simulink model "B_dot_filter"  (R2023a)
settings: Solver=ode45  StartTime=0.0  StopTime=48000.0  RelTol=1e-3  EnableMultiTasking=on
libraries: aausat3_lib x5
settings Model: NumberOfSteps=1000  Creator=KFJensen  LastModifiedBy=jacobel-omar
settings SolverCC: AlgebraicLoopSolver=TrustRegion
settings DataIOCC: SaveFormat=Array  SignalLoggingSaveFormat=ModelDataLogs  ReturnWorkspaceOutputs=off
settings OptimizationCC: DefaultParameterBehavior=Inlined  ExpressionDepthLimit=2147483647  LifeSpan=inf  SimCompilerOptimization=on
settings DebuggingCC: SignalInfNanChecking=error  UnderspecifiedInitializationDetection=Classic  MergeDetectMultiDrivingBlocksExec=none  SolverPrmCheckMsg=warning  IntegerOverflowMsg=error  ParameterUnderflowMsg=error  FcnCallInpInsideContextMsg=warning  UnconnectedInputMsg=warning  UnconnectedOutputMsg=warning  UnconnectedLineMsg=warning  AssertControl=DisableAll  StateNameClashWarn=warning  SFUnexpectedBacktrackingDiag=warning  SFNoUnconditionalDefaultTransitionDiag=warning  SFExecutionAtInitializationDiag=none  IntegerSaturationMsg=error  ArithmeticOperatorsInVariantConditions=warning
settings HardwareCC: ProdBitPerPointer=32  ProdBitPerSizeT=32  ProdBitPerPtrDiffT=32  ProdLargestAtomicFloat=None  ProdIntDivRoundTo=Undefined  ProdEndianess=Unspecified  ProdWordSize=32  ProdHWDeviceType=Generic->Unspecified (assume 32-bit Generic)
settings ModelReferenceCC: PropagateSignalLabelsOutOfModel=off
settings SFSimCC: SimUseLocalCustomCode=off  SimParseCustomCode=off  CustomCodeUndefinedFunction=UseInterfaceOnly
settings RTWCC: RTWUseLocalCustomCode=off
settings CodeAppCC: StateflowObjectComments=on
settings GRTTargetCC: TargetLangStandard=C89/C90 (ANSI)  CombineOutputUpdateFcns=off  GRTInterface=on
settings ConfigComp: CovMetricSettings=dw  CovSaveCumulativeToWorkspaceVar=on  CovSaveSingleToWorkspaceVar=on  CovExternalEMLEnable=off

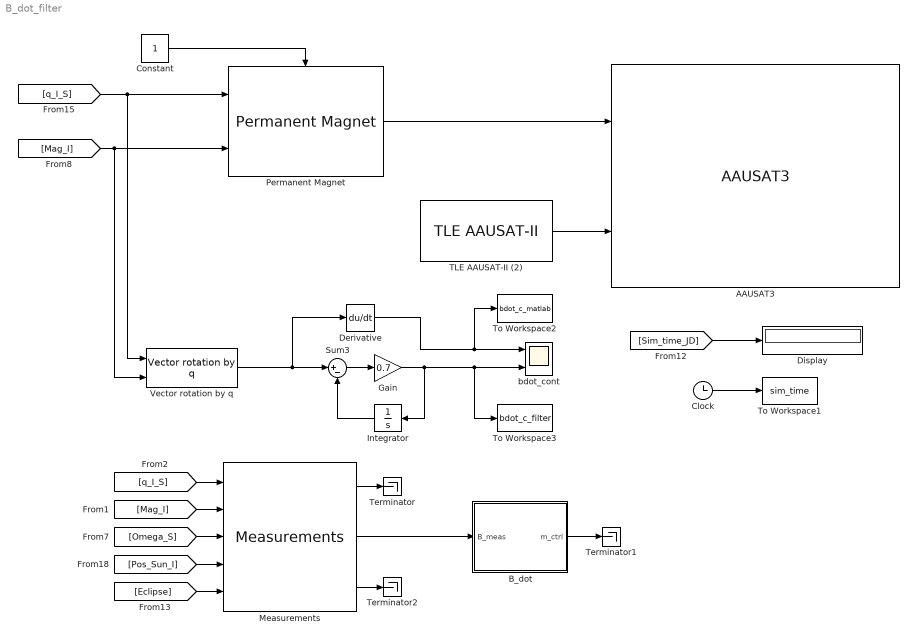
== system B_dot_filter ==
  AAUSAT3 : aausat3_lib/AAUSAT3  r_com_s=[0.049073,0.048909,0.042976]  sat_temp_start=293.15  mass_sc=0.957820  Dim=[0.1,0.1,0.11]  inertia_c=[0.0017464,0.0022092,0.0022388]  init_jd=2455153.1954318  q_s_c=[-0.020656,0.71468,-0.007319,0.6991]  q_init_I_S=[1 0 0 0]  w_init_s=[1,1,1]*10*pi/180  Cd=2  rho=5e-14  solar_m_flux=4.5565e-6  solar_absorb_coeff=1.5  theta_e=65  refldata=load('lib/AlbedoToolbox-1.0/refl_data/2005/ga050101-051231')  redfac=1  Ts=1  enable_sensor_emulation=on  enable_env_disturbance=on
      settings: SourceProductName=AAUSAT3
  B_dot : Subsystem  AncestorBlock=aausat3_lib/ACS/B_dot  mask{C=6000, wc=0.7, m_pm=-0.0030, Ts=0.1}
      mask prompts: C "Gain:"; wc "Filter cutoff frequency:"; m_pm "Permanent magnet dipole moment:"; Ts "Sample time:"
  Clock : Clock
  Constant : Constant
  Derivative : Derivative
  Display : Display
  Gain : Gain  Gain=0.7
  Integrator : Integrator
  Measurements : aausat3_lib/Sensor Emulation/Measurements  s_freq_mag=10  noise_mag=3  bias_mag=[0 0 0]  heading_mag=0  tilt_mag=0  s_freq_sun=1  noise_sun=3.33  bias_sun=[0 0]  nr_sample_sun=1  s_freq_gyro=1  noise_gyro=0.2  bias_gyro=[0 0 0]  heading_gyro=0  tilt_gyro=0
      settings: SourceProductName=AAUSAT3
  Permanent Magnet : aausat3_lib/Actuator Emulation/Permanent Magnet  mag_moment=-0.0030
      settings: SourceProductName=AAUSAT3
  Sum3 : Sum  Inputs=|+-
  TLE AAUSAT-II (2) : aausat3_lib/Orbit and Ephemeris/TLE AAUSAT-II  satname='AAUSAT-II'  JulianDay=09321.69542252  xndt2o=0.00000555  xndd6o=0.0  bstar=.76898e-4  xincl=97.9251  xnodeo=24.1597  eo=0.0014245  omegao=254.1774  xmo=105.7862  xno=14.81823818  ts=1
      settings: SourceProductName=AAUSAT3
  Terminator : Terminator
  Terminator1 : Terminator
  Terminator2 : Terminator
  To Workspace1 : ToWorkspace  VariableName=sim_time  SampleTime=-1
  To Workspace2 : ToWorkspace  VariableName=bdot_c_matlab  SampleTime=-1
  To Workspace3 : ToWorkspace  VariableName=bdot_c_filter  SampleTime=-1
  Vector rotation by q : aausat3_lib/Actuator Emulation/Permanent Magnet/Vector rotation by q  SystemSampleTime=-1  VariantActivationTime=update diagram  Latency=0  AutoFrameSizeCalculation=off
      settings: SourceProductName=AAUSAT3
  bdot_cont : Scope  NumInputPorts=2
  wires:
  TLE AAUSAT-II (2)/1 -> AAUSAT3/2
  [q_I_S] -> Permanent Magnet/1, Vector rotation by q/1
  [Mag_I] -> Permanent Magnet/2, Vector rotation by q/2
  Constant/1 -> Permanent Magnet/Enable
  [q_I_S] -> Measurements/1
  [Mag_I] -> Measurements/2
  [Omega_S] -> Measurements/3
  [Sim_time_JD] -> Display/1
  [Eclipse] -> Measurements/5
  [Pos_Sun_I] -> Measurements/4
  Measurements/1 -> Terminator/1
  Measurements/3 -> Terminator2/1
  Permanent Magnet/1 -> AAUSAT3/1
  Vector rotation by q/1 -> Sum3/1, Derivative/1
  Integrator/1 -> Sum3/2
  Sum3/1 -> Gain/1
  Gain/1 -> Integrator/1, bdot_cont/2, To Workspace3/1
  Derivative/1 -> bdot_cont/1, To Workspace2/1
  Measurements/2 -> B_dot/1(B_meas)
  B_dot/1(m_ctrl) -> Terminator1/1
  Clock/1 -> To Workspace1/1

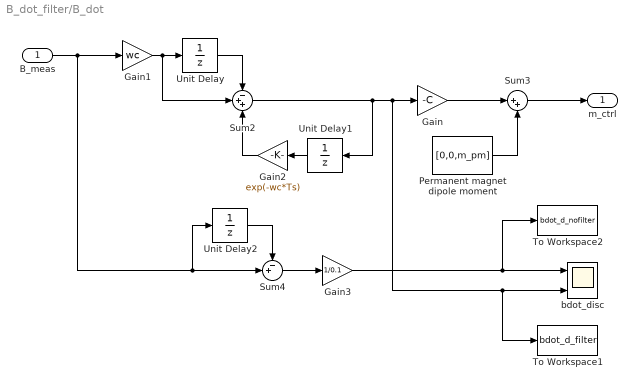
== system B_dot_filter/B_dot ==
  B_meas : Inport
  Gain : Gain  Gain=-C
  Gain1 : Gain  Gain=wc
  Gain2 : Gain  Gain=exp(-wc*Ts)
  Gain3 : Gain  Gain=1/0.1
  Permanent magnet dipole moment : Constant  Value=[0,0,m_pm]
  Sum2 : Sum  Inputs=-++
  Sum3 : Sum  Inputs=|++
  Sum4 : Sum  Inputs=-+|
  To Workspace1 : ToWorkspace  VariableName=bdot_d_filter  SampleTime=-1
  To Workspace2 : ToWorkspace  VariableName=bdot_d_nofilter  SampleTime=-1
  Unit Delay : UnitDelay  SampleTime=-1
  Unit Delay1 : UnitDelay  SampleTime=-1
  Unit Delay2 : UnitDelay  SampleTime=-1
  bdot_disc : Scope  NumInputPorts=2
  m_ctrl : Outport  PortDimensions=3
  wires:
  Sum3/1 -> m_ctrl/1
  Gain/1 -> Sum3/1
  Permanent magnet dipole moment/1 -> Sum3/2
  Sum2/1 -> Unit Delay1/1, Gain/1, bdot_disc/2, To Workspace1/1
  Unit Delay1/1 -> Gain2/1
  Gain2/1 -> Sum2/3
  Gain1/1 -> Sum2/2, Unit Delay/1
  Unit Delay/1 -> Sum2/1
  B_meas/1 -> Gain1/1, Sum4/2, Unit Delay2/1
  Unit Delay2/1 -> Sum4/1
  Sum4/1 -> Gain3/1
  Gain3/1 -> bdot_disc/1, To Workspace2/1
